simulink model "Lab1Simulink"  (R2014a)
settings: Solver=ode45  StartTime=0.0  StopTime=10.0  RelTol=1e-3
settings Model: Creator=User  LastModifiedBy=User

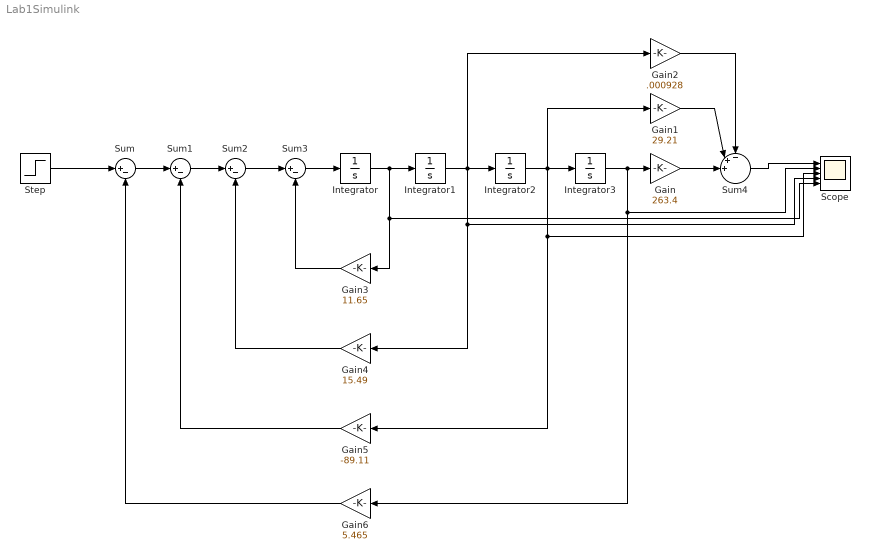
== system Lab1Simulink ==
  Gain : Gain  Gain=263.4
  Gain1 : Gain  Gain=29.21
  Gain2 : Gain  Gain=.000928
  Gain3 : Gain  Gain=11.65
  Gain4 : Gain  Gain=15.49
  Gain5 : Gain  Gain=-89.11
  Gain6 : Gain  Gain=5.465
  Integrator{,1..3} (4 alike) : Integrator
  Scope : Scope  NumInputPorts=5
      settings: YMin=-5~-5~-5~-5~-5  YMax=5~5~5~5~5
  Step : Step  SampleTime=0
  Sum{,1..3} (4 alike) : Sum  Inputs=|+-
  Sum4 : Sum  Inputs=-++||
  wires:
  Sum3/1 -> Integrator/1
  Integrator/1 -> Scope/5, Gain3/1, Integrator1/1
  Integrator1/1 -> Gain4/1, Scope/4, Gain2/1, Integrator2/1
  Integrator3/1 -> Scope/2, Gain6/1, Gain/1
  Gain1/1 -> Sum4/2
  Gain2/1 -> Sum4/1
  Gain3/1 -> Sum3/2
  Gain4/1 -> Sum2/2
  Gain5/1 -> Sum1/2
  Gain6/1 -> Sum/2
  Sum/1 -> Sum1/1
  Sum1/1 -> Sum2/1
  Sum2/1 -> Sum3/1
  Step/1 -> Sum/1
  Gain/1 -> Sum4/3
  Integrator2/1 -> Scope/3, Gain5/1, Gain1/1, Integrator3/1
  Sum4/1 -> Scope/1
